simulink model "controller_dev_sg_HIL_noTP"  (R2018b)
settings: configuration reference "Physics" (kept outside this file)
model workspace (MAT data in the model file):
  m = 1000
values from neighbouring files (symbols this model uses):
  bool_activate_Vehicles : value not decoded    [controller_dev_sg.sldd]
  ModObj_ObjList_SendPort = 11004.0    [UDPPortConfig.sldd]
  ModSens_GpsSenDat_SendPort = 3002.0    [UDPPortConfig.sldd]
  sensors_freq_camera = 37.0    [controller_dev_sg.sldd]
  sensors_freq_gps = 20.0    [controller_dev_sg.sldd]
  sensors_freq_imu = 100.0    [controller_dev_sg.sldd]
  sensors_freq_lidar = 12.0    [controller_dev_sg.sldd]
  sensors_freq_radar = 20.0    [controller_dev_sg.sldd]
undefined symbols (not defined in the file or in its folder): activate_VariableFriction, C, tpa_map_Reference, tSPhysics, x0_vehiclepos_start_veh1, x0_vehiclepos_start_veh10, x0_vehiclepos_start_veh2, x0_vehiclepos_start_veh3, x0_vehiclepos_start_veh4, x0_vehiclepos_start_veh5, x0_vehiclepos_start_veh6, x0_vehiclepos_start_veh7, x0_vehiclepos_start_veh8, x0_vehiclepos_start_veh9
libraries: xpcutilitieslib x273, xpcrtudplib x215, aerolibconvert2 x48, simulink x30, etargetslib x26, speedgoatlib_IO612 x7, canmsglib x6, slrtlib x4
(part 13 of 16)

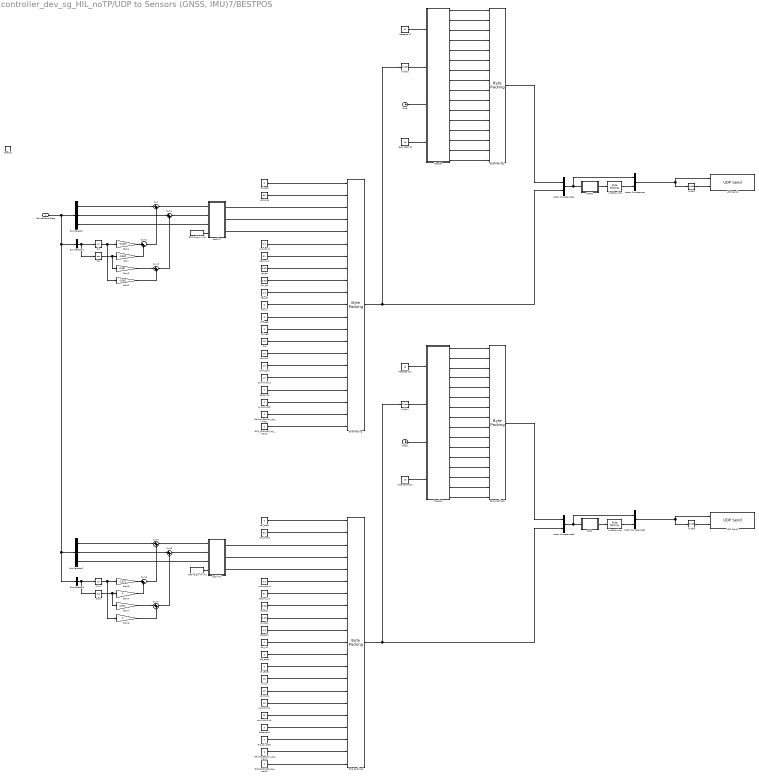
== system controller_dev_sg_HIL_noTP/UDP to Sensors (GNSS, IMU)7/BESTPOS ==
  VehicleSensorData : Inport
  Enable : EnablePort
  Bus Selector : BusSelector  OutputSignals=x_Loc1_m,y_Loc1_m,z_Loc1_m
  Bus Selector1 : BusSelector  OutputSignals=psi_YawAngleLoc1_rad
  Bus Selector2 : BusSelector  OutputSignals=x_Loc1_m,y_Loc1_m,z_Loc1_m
  Bus Selector3 : BusSelector  OutputSignals=psi_YawAngleLoc1_rad
  Byte Packing{,1..3} (4 alike) : xpcutilitieslib/Byte Packing 
  CRC1 : MATLAB Function  TreatAsAtomicUnit=on
  CRC32 : MATLAB Function  TreatAsAtomicUnit=on
  Clock : Clock
  Clock1 : Clock
  Cos : Trigonometry  Operator=cos
  Cos1 : Trigonometry  Operator=cos
  GPS Origin in llh : Constant  Value=[39.809786; -86.235148; 0.0]  OutDataTypeStr=double
  GPS Origin in llh1 : Constant  Value=[39.809786; -86.235148; 0.0]  OutDataTypeStr=double
  GPS_GLONASS_sig_mask1 : Constant  Value=0  OutDataTypeStr=uint8
  GPS_GLONASS_sig_mask2 : Constant  Value=0  OutDataTypeStr=uint8
  Gain : Gain  Gain=-0.502
  Gain1 : Gain  Gain=-0.457
  Gain2 : Gain  Gain=-0.502
  Gain3 : Gain  Gain=0.457
  Gain4 : Gain  Gain=0
  Gain5 : Gain  Gain=-1.571
  Gain6 : Gain  Gain=0
  Gain7 : Gain  Gain=1.571
  Galileo_BeiDou_sig_mask : Constant  Value=6  OutDataTypeStr=uint8
  Galileo_BeiDou_sig_mask1 : Constant  Value=6  OutDataTypeStr=uint8
  Header : MATLAB Function  TreatAsAtomicUnit=on
  Header1 : MATLAB Function  TreatAsAtomicUnit=on
  Message ID : Constant  Value=42  OutDataTypeStr=uint16
  Message ID1 : Constant  Value=42  OutDataTypeStr=uint16
  Reserved : Constant  Value=0  OutDataTypeStr=uint8
  Reserved1 : Constant  Value=0  OutDataTypeStr=uint8
  SVs : Constant  Value=19  OutDataTypeStr=uint8
  SVs1 : Constant  Value=19  OutDataTypeStr=uint8
  Sin : Trigonometry
  Sin1 : Trigonometry
  Sum{,1..7} (8 alike) : Sum  Inputs=|++
  UDP Send1 : xpcrtudplib/UDP Send  ipAddressVal=10.0.0.20  localPort=40681  toAddress=10.0.0.18  toPort=ModSens_GpsSenDat_SendPort  sampleTime=-1
      settings: SourceProductName=Simulink Real-Time  SourceProductBaseCode=XP
  UDP Send2 : xpcrtudplib/UDP Send  ipAddressVal=10.0.0.20  localPort=40781  toAddress=10.0.0.18  toPort=ModSens_GpsSenDat_SendPort + 1  sampleTime=-1
      settings: SourceProductName=Simulink Real-Time  SourceProductBaseCode=XP
  Vector Concatenate{,1..3} (4 alike) : Concatenate
  Width{1..4} (4 alike) : Width
  datum_id : Constant  Value=61  OutDataTypeStr=uint32
  datum_id1 : Constant  Value=61  OutDataTypeStr=uint32
  diff_age : Constant  Value=0  OutDataTypeStr=single
  diff_age1 : Constant  Value=0  OutDataTypeStr=single
  ext_sol_stat : Constant  Value=0  OutDataTypeStr=uint8
  ext_sol_stat1 : Constant  Value=0  OutDataTypeStr=uint8
  hgt_std : Constant  Value=1.0  OutDataTypeStr=single
  hgt_std1 : Constant  Value=1.0  OutDataTypeStr=single
  lat_std : Constant  Value=0.05  OutDataTypeStr=single
  lat_std1 : Constant  Value=0.05  OutDataTypeStr=single
  leap seconds : Constant  Value=19  OutDataTypeStr=single
  leap seconds1 : Constant  Value=19  OutDataTypeStr=single
  lon_std : Constant  Value=0.05  OutDataTypeStr=single
  lon_std1 : Constant  Value=0.05  OutDataTypeStr=single
  pos_type : Constant  Value=50  OutDataTypeStr=uint32
  pos_type1 : Constant  Value=50  OutDataTypeStr=uint32
  sol_age : Constant  Value=0  OutDataTypeStr=single
  sol_age1 : Constant  Value=0  OutDataTypeStr=single
  sol_stat : Constant  Value=0  OutDataTypeStr=uint32
  sol_stat1 : Constant  Value=0  OutDataTypeStr=uint32
  solnL1SVs : Constant  Value=19  OutDataTypeStr=uint8
  solnL1SVs1 : Constant  Value=19  OutDataTypeStr=uint8
  solnMultiSVs : Constant  Value=19  OutDataTypeStr=uint8
  solnMultiSVs1 : Constant  Value=19  OutDataTypeStr=uint8
  solnSVs : Constant  Value=19  OutDataTypeStr=uint8
  solnSVs1 : Constant  Value=19  OutDataTypeStr=uint8
  stn_id : Constant  Value=0  OutDataTypeStr=uint32
  stn_id1 : Constant  Value=0  OutDataTypeStr=uint32
  tcs2llhT : MATLAB Function  TreatAsAtomicUnit=on
  tcs2llhT1 : MATLAB Function  TreatAsAtomicUnit=on
  uint32touint1 : xpcutilitieslib/Byte Packing   MaskPackedDataType=uint8  MaskUnpackedDataTypes={'uint32'}  MaskAlignment=1
  uint32touint8 : xpcutilitieslib/Byte Packing   MaskPackedDataType=uint8  MaskUnpackedDataTypes={'uint32'}  MaskAlignment=1
  undulation : Constant  Value=0.0  OutDataTypeStr=single
  undulation1 : Constant  Value=0.0  OutDataTypeStr=single
  wires:
  CRC32/1(crc) -> uint32touint8/1
  uint32touint8/1 -> Vector Concatenate/2
  sol_stat/1 -> Byte Packing/1
  pos_type/1 -> Byte Packing/2
  undulation/1 -> Byte Packing/6
  datum_id/1 -> Byte Packing/7
  lat_std/1 -> Byte Packing/8
  lon_std/1 -> Byte Packing/9
  hgt_std/1 -> Byte Packing/10
  stn_id/1 -> Byte Packing/11
  diff_age/1 -> Byte Packing/12
  sol_age/1 -> Byte Packing/13
  SVs/1 -> Byte Packing/14
  solnSVs/1 -> Byte Packing/15
  solnL1SVs/1 -> Byte Packing/16
  solnMultiSVs/1 -> Byte Packing/17
  Reserved/1 -> Byte Packing/18
  ext_sol_stat/1 -> Byte Packing/19
  Galileo_BeiDou_sig_mask/1 -> Byte Packing/20
  GPS_GLONASS_sig_mask1/1 -> Byte Packing/21
  Header/1(first) -> Byte Packing1/1
  Header/2(second) -> Byte Packing1/2
  Header/3(third) -> Byte Packing1/3
  Header/4(hlength) -> Byte Packing1/4
  Header/5(id) -> Byte Packing1/5
  Header/6(type) -> Byte Packing1/6
  Header/7(port) -> Byte Packing1/7
  Header/8(mlength) -> Byte Packing1/8
  Header/9(seq) -> Byte Packing1/9
  Header/10(idletime) -> Byte Packing1/10
  Header/11(timestatus) -> Byte Packing1/11
  Header/12(week) -> Byte Packing1/12
  Header/13(ms) -> Byte Packing1/13
  Header/14(recstatus) -> Byte Packing1/14
  Header/15(reserved) -> Byte Packing1/15
  Header/16(version) -> Byte Packing1/16
  Message ID/1 -> Header/1("id ")
  Width2/1 -> Header/2(length)
  leap seconds/1 -> Header/4(leapseconds)
  Clock/1 -> Header/3(time)
  Vector Concatenate1/1 -> Vector Concatenate/1, CRC32/1(data)
  Byte Packing1/1 -> Vector Concatenate1/1
  Byte Packing/1 -> Width2/1, Vector Concatenate1/2
  Bus Selector/3 -> tcs2llhT/3(z)  "<z_Loc1_m>"
  tcs2llhT/1(lat) -> Byte Packing/3
  tcs2llhT/2(lon) -> Byte Packing/4
  tcs2llhT/3(hgt) -> Byte Packing/5
  GPS Origin in llh/1 -> tcs2llhT/4(origin)
  Width1/1 -> UDP Send1/2
  Vector Concatenate/1 -> UDP Send1/1, Width1/1
  Bus Selector/1 -> Sum/1  "<x_Loc1_m>"
  Bus Selector/2 -> Sum1/1  "<y_Loc1_m>"
  Sum1/1 -> tcs2llhT/2(y)
  Sum/1 -> tcs2llhT/1(x)
  Bus Selector1/1 -> Cos/1, Sin/1  "<psi_YawAngleLoc1_rad>"
  Cos/1 -> Gain3/1, Gain/1
  Sin/1 -> Gain2/1, Gain1/1
  Gain1/1 -> Sum2/1
  Gain/1 -> Sum2/2
  Sum2/1 -> Sum/2
  Gain2/1 -> Sum3/2
  Gain3/1 -> Sum3/1
  Sum3/1 -> Sum1/2
  Sum7/1 -> Sum5/2
  Gain4/1 -> Sum6/2
  Gain5/1 -> Sum6/1
  Sum6/1 -> Sum4/2
  Sin1/1 -> Gain6/1, Gain5/1
  Cos1/1 -> Gain7/1, Gain4/1
  Bus Selector3/1 -> Cos1/1, Sin1/1  "<psi_YawAngleLoc1_rad>"
  Header1/1(first) -> Byte Packing3/1
  lon_std1/1 -> Byte Packing2/9
  Header1/10(idletime) -> Byte Packing3/10
  tcs2llhT1/2(lon) -> Byte Packing2/4
  Header1/8(mlength) -> Byte Packing3/8
  tcs2llhT1/3(hgt) -> Byte Packing2/5
  tcs2llhT1/1(lat) -> Byte Packing2/3
  Header1/5(id) -> Byte Packing3/5
  undulation1/1 -> Byte Packing2/6
  Header1/9(seq) -> Byte Packing3/9
  Width4/1 -> Header1/2(length)
  Byte Packing2/1 -> Width4/1, Vector Concatenate3/2
  GPS Origin in llh1/1 -> tcs2llhT1/4(origin)
  Header1/2(second) -> Byte Packing3/2
  Header1/4(hlength) -> Byte Packing3/4
  Header1/3(third) -> Byte Packing3/3
  Header1/16(version) -> Byte Packing3/16
  Header1/6(type) -> Byte Packing3/6
  SVs1/1 -> Byte Packing2/14
  datum_id1/1 -> Byte Packing2/7
  Vector Concatenate3/1 -> Vector Concatenate2/1, CRC1/1(data)
  Clock1/1 -> Header1/3(time)
  Header1/11(timestatus) -> Byte Packing3/11
  leap seconds1/1 -> Header1/4(leapseconds)
  Header1/7(port) -> Byte Packing3/7
  stn_id1/1 -> Byte Packing2/11
  VehicleSensorData/1 -> Bus Selector3/1, Bus Selector2/1, Bus Selector1/1, Bus Selector/1
  lat_std1/1 -> Byte Packing2/8
  solnMultiSVs1/1 -> Byte Packing2/17
  pos_type1/1 -> Byte Packing2/2
  Vector Concatenate2/1 -> UDP Send2/1, Width3/1
  solnL1SVs1/1 -> Byte Packing2/16
  Bus Selector2/3 -> tcs2llhT1/3(z)  "<z_Loc1_m>"
  solnSVs1/1 -> Byte Packing2/15
  Message ID1/1 -> Header1/1("id ")
  Header1/15(reserved) -> Byte Packing3/15
  sol_age1/1 -> Byte Packing2/13
  Header1/12(week) -> Byte Packing3/12
  uint32touint1/1 -> Vector Concatenate2/2
  CRC1/1(crc) -> uint32touint1/1
  GPS_GLONASS_sig_mask2/1 -> Byte Packing2/21
  Byte Packing3/1 -> Vector Concatenate3/1
  Reserved1/1 -> Byte Packing2/18
  Sum5/1 -> tcs2llhT1/2(y)
  Header1/14(recstatus) -> Byte Packing3/14
  diff_age1/1 -> Byte Packing2/12
  sol_stat1/1 -> Byte Packing2/1
  Header1/13(ms) -> Byte Packing3/13
  Galileo_BeiDou_sig_mask1/1 -> Byte Packing2/20
  Bus Selector2/2 -> Sum5/1  "<y_Loc1_m>"
  Gain7/1 -> Sum7/1
  Sum4/1 -> tcs2llhT1/1(x)
  Bus Selector2/1 -> Sum4/1  "<x_Loc1_m>"
  Gain6/1 -> Sum7/2
  ext_sol_stat1/1 -> Byte Packing2/19
  hgt_std1/1 -> Byte Packing2/10
  Width3/1 -> UDP Send2/2

== system controller_dev_sg_HIL_noTP/UDP to Sensors (GNSS, IMU)7/BESTUTM ==
  VehicleSensorData : Inport
  Enable : EnablePort
  Bus Selector : BusSelector  OutputSignals=x_Loc1_m,y_Loc1_m,z_Loc1_m
  Byte Packing : xpcutilitieslib/Byte Packing   MaskPackedDataType=uint8  MaskUnpackedDataTypes={'uint32', 'uint32', 'uint32', 'uint32', 'double', 'double', 'double', 'single', 'uint32', 'single', 'single', 'single', 'uint32', 'single', 'single', 'uint8', 'uint8', 'uint8', 'uint8', 'uint8', 'uint8', 'uint8', 'uint8'}  MaskAlignment=1
  Byte Packing1 : xpcutilitieslib/Byte Packing   MaskPackedDataType=uint8  MaskUnpackedDataTypes={'uint8', 'uint8', 'uint8', 'uint8', 'uint16', 'uint8', 'uint8', 'uint16', 'uint16', 'uint8', 'uint8', 'uint16', 'uint32', 'uint32', 'uint16', 'uint16'}  MaskAlignment=1
  CRC32 : MATLAB Function  TreatAsAtomicUnit=on
  Clock : Clock
  Data Type Conversion : DataTypeConversion  OutDataTypeStr=uint32
  Data Type Conversion1 : DataTypeConversion  OutDataTypeStr=uint32
  GPS Origin in llh : Constant  Value=[39.809786; -86.235148; 0.0]  OutDataTypeStr=double
  GPS_GLONASS_sig_mask1 : Constant  Value=0  OutDataTypeStr=uint8
  Galileo_BeiDou_sig_mask : Constant  Value=6  OutDataTypeStr=uint8
  Header : MATLAB Function  TreatAsAtomicUnit=on
  MATLAB Function : MATLAB Function  TreatAsAtomicUnit=on
  Message ID : Constant  Value=726  OutDataTypeStr=uint16
  Reserved : Constant  Value=0  OutDataTypeStr=uint8
  SVs : Constant  Value=19  OutDataTypeStr=uint8
  UDP Send1 : xpcrtudplib/UDP Send  ipAddressVal=10.0.0.20  localPort=40785  toAddress=10.0.0.18  toPort=ModSens_GpsSenDat_SendPort + 1  sampleTime=-1
      settings: SourceProductName=Simulink Real-Time  SourceProductBaseCode=XP
  UDP Send5 : xpcrtudplib/UDP Send  ipAddressVal=10.0.0.20  localPort=40685  toAddress=10.0.0.18  toPort=ModSens_GpsSenDat_SendPort  sampleTime=-1
      settings: SourceProductName=Simulink Real-Time  SourceProductBaseCode=XP
  Vector Concatenate : Concatenate
  Vector Concatenate1 : Concatenate
  Width2 : Width
  Width5 : Width
  datum id : Constant  Value=61  OutDataTypeStr=uint32
  diff_age : Constant  Value=0  OutDataTypeStr=single
  e std : Constant  Value=0  OutDataTypeStr=single
  ext sol stat : Constant  Value=0  OutDataTypeStr=uint8
  ggL1 : Constant  Value=19  OutDataTypeStr=uint8
  hgt std : Constant  Value=0  OutDataTypeStr=single
  leap seconds : Constant  Value=19  OutDataTypeStr=single
  n std : Constant  Value=0  OutDataTypeStr=single
  pos_type : Constant  Value=16  OutDataTypeStr=uint32
  sol_age : Constant  Value=0  OutDataTypeStr=single
  sol_stat : Constant  Value=0  OutDataTypeStr=uint32
  solnMultiSV : Constant  Value=19  OutDataTypeStr=uint8
  solnSVs : Constant  Value=19  OutDataTypeStr=uint8
  stn id : Constant  Value=0  OutDataTypeStr=uint32
  tcs2llhT : MATLAB Function  TreatAsAtomicUnit=on
  uint32touint8 : xpcutilitieslib/Byte Packing   MaskPackedDataType=uint8  MaskUnpackedDataTypes={'uint32'}  MaskAlignment=1
  undulation : Constant  Value=0.0  OutDataTypeStr=single
  wires:
  VehicleSensorData/1 -> Bus Selector/1
  CRC32/1(crc) -> uint32touint8/1
  uint32touint8/1 -> Vector Concatenate/2
  Message ID/1 -> Header/1("id ")
  Header/7(port) -> Byte Packing1/7
  Byte Packing1/1 -> Vector Concatenate1/1
  Header/9(seq) -> Byte Packing1/9
  Width2/1 -> Header/2(length)
  Header/12(week) -> Byte Packing1/12
  Header/1(first) -> Byte Packing1/1
  leap seconds/1 -> Header/4(leapseconds)
  Header/4(hlength) -> Byte Packing1/4
  Header/8(mlength) -> Byte Packing1/8
  Header/10(idletime) -> Byte Packing1/10
  Header/2(second) -> Byte Packing1/2
  Header/15(reserved) -> Byte Packing1/15
  Clock/1 -> Header/3(time)
  Header/14(recstatus) -> Byte Packing1/14
  Header/6(type) -> Byte Packing1/6
  Header/5(id) -> Byte Packing1/5
  Header/3(third) -> Byte Packing1/3
  Header/16(version) -> Byte Packing1/16
  Header/13(ms) -> Byte Packing1/13
  Header/11(timestatus) -> Byte Packing1/11
  sol_stat/1 -> Byte Packing/1
  pos_type/1 -> Byte Packing/2
  undulation/1 -> Byte Packing/8
  datum id/1 -> Byte Packing/9
  n std/1 -> Byte Packing/10
  e std/1 -> Byte Packing/11
  hgt std/1 -> Byte Packing/12
  stn id/1 -> Byte Packing/13
  diff_age/1 -> Byte Packing/14
  sol_age/1 -> Byte Packing/15
  SVs/1 -> Byte Packing/16
  solnSVs/1 -> Byte Packing/17
  ggL1/1 -> Byte Packing/18
  solnMultiSV/1 -> Byte Packing/19
  Reserved/1 -> Byte Packing/20
  ext sol stat/1 -> Byte Packing/21
  Galileo_BeiDou_sig_mask/1 -> Byte Packing/22
  GPS_GLONASS_sig_mask1/1 -> Byte Packing/23
  Vector Concatenate1/1 -> Vector Concatenate/1, CRC32/1(data)
  Byte Packing/1 -> Width2/1, Vector Concatenate1/2
  GPS Origin in llh/1 -> tcs2llhT/4(origin)
  tcs2llhT/3(hgt) -> Byte Packing/7
  Bus Selector/2 -> tcs2llhT/2(y)  "<y_Loc1_m>"
  Bus Selector/1 -> tcs2llhT/1(x)  "<x_Loc1_m>"
  Bus Selector/3 -> tcs2llhT/3(z)  "<z_Loc1_m>"
  tcs2llhT/1(lat) -> MATLAB Function/1(Lat)
  tcs2llhT/2(lon) -> MATLAB Function/2(Lon)
  MATLAB Function/1(zone_nbr) -> Data Type Conversion/1
  Data Type Conversion/1 -> Byte Packing/3
  MATLAB Function/2(zone_ltr) -> Data Type Conversion1/1
  Data Type Conversion1/1 -> Byte Packing/4
  MATLAB Function/3(northing) -> Byte Packing/5
  MATLAB Function/4(easting) -> Byte Packing/6
  Vector Concatenate/1 -> UDP Send1/1, UDP Send5/1, Width5/1
  Width5/1 -> UDP Send1/2, UDP Send5/2

== system controller_dev_sg_HIL_noTP/UDP to Sensors (GNSS, IMU)7/BESTVAL ==
  VehicleSensorData : Inport
  SimRealState : Inport  Port=2
  Enable : EnablePort
  Angle Conversion2 : aerolibconvert2/Angle Conversion  IU=rad  OU=deg
  Bus Selector : BusSelector  OutputSignals=vx_CoGVel1_mps,vy_CoGVel1_mps,x_Loc1_m,y_Loc1_m,z_Loc1_m
  Bus Selector1 : BusSelector  OutputSignals=psi_rad
  Byte Packing : xpcutilitieslib/Byte Packing   MaskPackedDataType=uint8  MaskUnpackedDataTypes={'uint32', 'uint32', 'single', 'single', 'double', 'double', 'double', 'single'}  MaskAlignment=1
  Byte Packing1 : xpcutilitieslib/Byte Packing   MaskPackedDataType=uint8  MaskUnpackedDataTypes={'uint8', 'uint8', 'uint8', 'uint8', 'uint16', 'uint8', 'uint8', 'uint16', 'uint16', 'uint8', 'uint8', 'uint16', 'uint32', 'uint32', 'uint16', 'uint16'}  MaskAlignment=1
  CRC32 : MATLAB Function  TreatAsAtomicUnit=on
  Clock : Clock
  GPS Origin in llh : Constant  Value=[39.809786; -86.235148; 0.0]  OutDataTypeStr=double
  Gain : Gain  Gain=-1
  Header : MATLAB Function  TreatAsAtomicUnit=on
  Message ID : Constant  Value=99  OutDataTypeStr=uint16
  Plus : Sum  AccumDataTypeStr=double
  Reserved : Constant  Value=0  OutDataTypeStr=single
  UDP Send1 : xpcrtudplib/UDP Send  ipAddressVal=10.0.0.20  localPort=40782  toAddress=10.0.0.18  toPort=ModSens_GpsSenDat_SendPort + 1  sampleTime=-1
      settings: SourceProductName=Simulink Real-Time  SourceProductBaseCode=XP
  UDP Send2 : xpcrtudplib/UDP Send  ipAddressVal=10.0.0.20  localPort=40682  toAddress=10.0.0.18  toPort=ModSens_GpsSenDat_SendPort  sampleTime=-1
      settings: SourceProductName=Simulink Real-Time  SourceProductBaseCode=XP
  Vector Concatenate : Concatenate
  Vector Concatenate1 : Concatenate
  Vector Concatenate2 : Concatenate
  Width1 : Width
  Width2 : Width
  age : Constant  Value=4  OutDataTypeStr=single
  grid conv angle : MATLAB Function  TreatAsAtomicUnit=on
  latency : Constant  Value=0.25  OutDataTypeStr=single
  leap seconds : Constant  Value=19  OutDataTypeStr=single
  norm : MATLAB Function  TreatAsAtomicUnit=on
  normalizeAngle360 : MATLAB Function  TreatAsAtomicUnit=on
  sol_stat : Constant  Value=0  OutDataTypeStr=uint32
  tcs2llhT : MATLAB Function  TreatAsAtomicUnit=on
  uint32touint8 : xpcutilitieslib/Byte Packing   MaskPackedDataType=uint8  MaskUnpackedDataTypes={'uint32'}  MaskAlignment=1
  vel_type : Constant  Value=17  OutDataTypeStr=uint32
  vert_spd : Constant  Value=0.0  OutDataTypeStr=double
  wires:
  VehicleSensorData/1 -> Bus Selector/1
  CRC32/1(crc) -> uint32touint8/1
  uint32touint8/1 -> Vector Concatenate/2
  Header/14(recstatus) -> Byte Packing1/14
  Header/15(reserved) -> Byte Packing1/15
  Header/16(version) -> Byte Packing1/16
  Header/13(ms) -> Byte Packing1/13
  Header/10(idletime) -> Byte Packing1/10
  Header/11(timestatus) -> Byte Packing1/11
  Clock/1 -> Header/3(time)
  Header/7(port) -> Byte Packing1/7
  Header/6(type) -> Byte Packing1/6
  Header/8(mlength) -> Byte Packing1/8
  Header/5(id) -> Byte Packing1/5
  Header/3(third) -> Byte Packing1/3
  Header/4(hlength) -> Byte Packing1/4
  Header/1(first) -> Byte Packing1/1
  leap seconds/1 -> Header/4(leapseconds)
  Message ID/1 -> Header/1("id ")
  Width2/1 -> Header/2(length)
  Header/2(second) -> Byte Packing1/2
  Header/12(week) -> Byte Packing1/12
  Byte Packing1/1 -> Vector Concatenate1/1
  Header/9(seq) -> Byte Packing1/9
  sol_stat/1 -> Byte Packing/1
  vel_type/1 -> Byte Packing/2
  latency/1 -> Byte Packing/3
  age/1 -> Byte Packing/4
  vert_spd/1 -> Byte Packing/7
  Reserved/1 -> Byte Packing/8
  Vector Concatenate1/1 -> Vector Concatenate/1, CRC32/1(data)
  Byte Packing/1 -> Width2/1, Vector Concatenate1/2
  Bus Selector/2 -> Vector Concatenate2/2  "<vy_CoGVel1_mps>"
  Bus Selector/1 -> Vector Concatenate2/1  "<vx_CoGVel1_mps>"
  Vector Concatenate2/1 -> norm/1(u)
  GPS Origin in llh/1 -> tcs2llhT/4(origin)
  Bus Selector/5 -> tcs2llhT/3(z)  "<z_Loc1_m>"
  Bus Selector/4 -> tcs2llhT/2(y)  "<y_Loc1_m>"
  Bus Selector/3 -> tcs2llhT/1(x)  "<x_Loc1_m>"
  tcs2llhT/1(lat) -> grid conv angle/1(lat)
  tcs2llhT/2(lon) -> grid conv angle/2(lon)
  norm/1(y) -> Byte Packing/5
  SimRealState/1 -> Bus Selector1/1
  Angle Conversion2/1 -> Gain/1
  Bus Selector1/1 -> Angle Conversion2/1  "<psi_rad>"
  Plus/1 -> normalizeAngle360/1(u)
  grid conv angle/1(gamma) -> Plus/1
  normalizeAngle360/1(y) -> Byte Packing/6
  Gain/1 -> Plus/2
  Vector Concatenate/1 -> Width1/1, UDP Send1/1, UDP Send2/1
  Width1/1 -> UDP Send1/2, UDP Send2/2

== system controller_dev_sg_HIL_noTP/UDP to Sensors (GNSS, IMU)7/CORRIMUDATA ==
  VehicleSensorData : Inport
  Enable : EnablePort
  Bus Selector : BusSelector  OutputSignals=dTheta_PitchRateIMU1_radps,dPhi_RollRateIMU1_radps,dPsi_YawRateIMU1_radps,ay_CoGIMU1_mps2,ax_CoGIMU1_mps2,az_CoGIMU1_mps2
  Byte Packing : xpcutilitieslib/Byte Packing   MaskPackedDataType=uint8  MaskUnpackedDataTypes={'uint32', 'double', 'double', 'double', 'double', 'double', 'double', 'double'}  MaskAlignment=1
  Byte Packing1 : xpcutilitieslib/Byte Packing   MaskPackedDataType=uint8  MaskUnpackedDataTypes={'uint8', 'uint8', 'uint8', 'uint8', 'uint16', 'uint8', 'uint8', 'uint16', 'uint16', 'uint8', 'uint8', 'uint16', 'uint32', 'uint32', 'uint16', 'uint16'}  MaskAlignment=1
  CRC32 : MATLAB Function  TreatAsAtomicUnit=on
  Clock : Clock
  Clock1 : Clock
  GNSS Week : Constant  Value=1900  OutDataTypeStr=uint32
  Header : MATLAB Function  TreatAsAtomicUnit=on
  Message ID : Constant  Value=812  OutDataTypeStr=uint16
  UDP Send1 : xpcrtudplib/UDP Send  ipAddressVal=10.0.0.20  localPort=40783  toAddress=10.0.0.18  toPort=ModSens_GpsSenDat_SendPort + 1  sampleTime=-1
      settings: SourceProductName=Simulink Real-Time  SourceProductBaseCode=XP
  UDP Send3 : xpcrtudplib/UDP Send  ipAddressVal=10.0.0.20  localPort=40683  toAddress=10.0.0.18  toPort=ModSens_GpsSenDat_SendPort  sampleTime=-1
      settings: SourceProductName=Simulink Real-Time  SourceProductBaseCode=XP
  Vector Concatenate : Concatenate
  Vector Concatenate1 : Concatenate
  Width2 : Width
  Width3 : Width
  leap seconds : Constant  Value=19  OutDataTypeStr=single
  uint32touint8 : xpcutilitieslib/Byte Packing   MaskPackedDataType=uint8  MaskUnpackedDataTypes={'uint32'}  MaskAlignment=1
  wires:
  VehicleSensorData/1 -> Bus Selector/1
  CRC32/1(crc) -> uint32touint8/1
  uint32touint8/1 -> Vector Concatenate/2
  Message ID/1 -> Header/1("id ")
  Header/9(seq) -> Byte Packing1/9
  Byte Packing1/1 -> Vector Concatenate1/1
  Header/12(week) -> Byte Packing1/12
  Width2/1 -> Header/2(length)
  leap seconds/1 -> Header/4(leapseconds)
  Header/2(second) -> Byte Packing1/2
  Header/6(type) -> Byte Packing1/6
  Header/4(hlength) -> Byte Packing1/4
  Header/8(mlength) -> Byte Packing1/8
  Header/5(id) -> Byte Packing1/5
  Header/1(first) -> Byte Packing1/1
  Header/3(third) -> Byte Packing1/3
  Header/16(version) -> Byte Packing1/16
  Header/11(timestatus) -> Byte Packing1/11
  Header/13(ms) -> Byte Packing1/13
  Header/10(idletime) -> Byte Packing1/10
  Header/15(reserved) -> Byte Packing1/15
  Header/14(recstatus) -> Byte Packing1/14
  Header/7(port) -> Byte Packing1/7
  Clock/1 -> Header/3(time)
  GNSS Week/1 -> Byte Packing/1
  Clock1/1 -> Byte Packing/2
  Vector Concatenate1/1 -> Vector Concatenate/1, CRC32/1(data)
  Byte Packing/1 -> Vector Concatenate1/2, Width2/1
  Bus Selector/1 -> Byte Packing/3  "<dTheta_PitchRateIMU1_radps>"
  Bus Selector/2 -> Byte Packing/4  "<dPhi_RollRateIMU1_radps>"
  Bus Selector/3 -> Byte Packing/5  "<dPsi_YawRateIMU1_radps>"
  Bus Selector/6 -> Byte Packing/8  "<az_CoGIMU1_mps2>"
  Bus Selector/4 -> Byte Packing/6  "<ay_CoGIMU1_mps2>"
  Bus Selector/5 -> Byte Packing/7  "<ax_CoGIMU1_mps2>"
  Width3/1 -> UDP Send1/2, UDP Send3/2
  Vector Concatenate/1 -> UDP Send1/1, UDP Send3/1, Width3/1

== system controller_dev_sg_HIL_noTP/UDP to Sensors (GNSS, IMU)7/DUALANTENNAHEADING ==
  VehicleSensorData : Inport
  SimRealState : Inport  Port=2
  Enable : EnablePort
  Angle Conversion{1..4} (4 alike) : aerolibconvert2/Angle Conversion  IU=rad  OU=deg
  Bus Selector : BusSelector  OutputSignals=x_Loc1_m,y_Loc1_m,z_Loc1_m,theta_PitchAngleLoc1_rad
  Bus Selector1 : BusSelector  OutputSignals=psi_rad
  Bus Selector2 : BusSelector  OutputSignals=x_Loc1_m,y_Loc1_m,z_Loc1_m,theta_PitchAngleLoc1_rad
  Bus Selector3 : BusSelector  OutputSignals=psi_rad
  Byte Packing{,1..3} (4 alike) : xpcutilitieslib/Byte Packing 
  CRC1 : MATLAB Function  TreatAsAtomicUnit=on
  CRC32 : MATLAB Function  TreatAsAtomicUnit=on
  Clock : Clock
  Clock1 : Clock
  Constant : Constant  Value=90  OutDataTypeStr=double
  Constant1 : Constant  Value=180  OutDataTypeStr=double
  Data Type Conversion{1..3,7} (4 alike) : DataTypeConversion  OutDataTypeStr=single
  GPS Origin in llh : Constant  Value=[39.809786; -86.235148; 0.0]  OutDataTypeStr=double
  GPS Origin in llh1 : Constant  Value=[39.809786; -86.235148; 0.0]  OutDataTypeStr=double
  GPS_GLONASS_sig_mask1 : Constant  Value=0  OutDataTypeStr=uint8
  GPS_GLONASS_sig_mask2 : Constant  Value=0  OutDataTypeStr=uint8
  Gain : Gain  Gain=-1
  Gain1 : Gain  Gain=-1
  Galileo_BeiDou_sig_mask : Constant  Value=6  OutDataTypeStr=uint8
  Galileo_BeiDou_sig_mask1 : Constant  Value=6  OutDataTypeStr=uint8
  Header : MATLAB Function  TreatAsAtomicUnit=on
  Header1 : MATLAB Function  TreatAsAtomicUnit=on
  Message ID : Constant  Value=2042  OutDataTypeStr=uint16
  Message ID1 : Constant  Value=2042  OutDataTypeStr=uint16
  Plus{,1..3} (4 alike) : Sum  AccumDataTypeStr=double
  Reserved : Constant  Value=0  OutDataTypeStr=single
  Reserved1 : Constant  Value=0  OutDataTypeStr=single
  SVs : Constant  Value=19  OutDataTypeStr=uint8
  SVs1 : Constant  Value=19  OutDataTypeStr=uint8
  UDP Send2 : xpcrtudplib/UDP Send  ipAddressVal=10.0.0.20  localPort=40788  toAddress=10.0.0.18  toPort=ModSens_GpsSenDat_SendPort + 1  sampleTime=-1
      settings: SourceProductName=Simulink Real-Time  SourceProductBaseCode=XP
  UDP Send3 : xpcrtudplib/UDP Send  ipAddressVal=10.0.0.20  localPort=40688  toAddress=10.0.0.18  toPort=ModSens_GpsSenDat_SendPort  sampleTime=-1
      settings: SourceProductName=Simulink Real-Time  SourceProductBaseCode=XP
  Vector Concatenate{,1..3} (4 alike) : Concatenate
  Width{1..4} (4 alike) : Width
  ext_sol_stat : Constant  Value=0  OutDataTypeStr=uint8
  ext_sol_stat1 : Constant  Value=0  OutDataTypeStr=uint8
  grid conv angle : MATLAB Function  TreatAsAtomicUnit=on
  grid conv angle1 : MATLAB Function  TreatAsAtomicUnit=on
  hdg std dev : Constant  Value=0  OutDataTypeStr=single
  hdg std dev1 : Constant  Value=0  OutDataTypeStr=single
  leap seconds : Constant  Value=19  OutDataTypeStr=single
  leap seconds1 : Constant  Value=19  OutDataTypeStr=single
  length : Constant  Value=-1  OutDataTypeStr=single
  length1 : Constant  Value=-1  OutDataTypeStr=single
  multi : Constant  Value=0  OutDataTypeStr=uint8
  multi1 : Constant  Value=0  OutDataTypeStr=uint8
  normalizeAngle1 : MATLAB Function  TreatAsAtomicUnit=on
  normalizeAngle360 : MATLAB Function  TreatAsAtomicUnit=on
  obs : Constant  Value=0  OutDataTypeStr=uint8
  obs1 : Constant  Value=0  OutDataTypeStr=uint8
  pos_type : Constant  Value=50  OutDataTypeStr=uint32
  pos_type1 : Constant  Value=50  OutDataTypeStr=uint32
  ptch std dev1 : Constant  Value=0  OutDataTypeStr=single
  ptch std dev2 : Constant  Value=0  OutDataTypeStr=single
  sol source : Constant  Value=0  OutDataTypeStr=uint8
  sol source1 : Constant  Value=0  OutDataTypeStr=uint8
  sol_stat : Constant  Value=0  OutDataTypeStr=uint32
  sol_stat1 : Constant  Value=0  OutDataTypeStr=uint32
  solnSVs : Constant  Value=19  OutDataTypeStr=uint8
  solnSVs1 : Constant  Value=19  OutDataTypeStr=uint8
  stn_id : Constant  Value=0  OutDataTypeStr=uint32
  stn_id1 : Constant  Value=0  OutDataTypeStr=uint32
  tcs2llhT : MATLAB Function  TreatAsAtomicUnit=on
  tcs2llhT1 : MATLAB Function  TreatAsAtomicUnit=on
  uint32touint1 : xpcutilitieslib/Byte Packing   MaskPackedDataType=uint8  MaskUnpackedDataTypes={'uint32'}  MaskAlignment=1
  uint32touint8 : xpcutilitieslib/Byte Packing   MaskPackedDataType=uint8  MaskUnpackedDataTypes={'uint32'}  MaskAlignment=1
  wires:
  CRC32/1(crc) -> uint32touint8/1
  uint32touint8/1 -> Vector Concatenate/2
  Vector Concatenate1/1 -> Vector Concatenate/1, CRC32/1(data)
  Width3/1 -> UDP Send3/2
  Vector Concatenate/1 -> UDP Send3/1, Width3/1
  Header/10(idletime) -> Byte Packing1/10
  Header/16(version) -> Byte Packing1/16
  Header/7(port) -> Byte Packing1/7
  Header/11(timestatus) -> Byte Packing1/11
  Header/8(mlength) -> Byte Packing1/8
  Header/12(week) -> Byte Packing1/12
  leap seconds/1 -> Header/4(leapseconds)
  Byte Packing1/1 -> Vector Concatenate1/1
  Header/6(type) -> Byte Packing1/6
  Header/9(seq) -> Byte Packing1/9
  Header/5(id) -> Byte Packing1/5
  Header/1(first) -> Byte Packing1/1
  Message ID/1 -> Header/1("id ")
  Width2/1 -> Header/2(length)
  Header/3(third) -> Byte Packing1/3
  Header/4(hlength) -> Byte Packing1/4
  Clock/1 -> Header/3(time)
  Header/2(second) -> Byte Packing1/2
  Header/15(reserved) -> Byte Packing1/15
  Byte Packing/1 -> Vector Concatenate1/2, Width2/1
  Header/14(recstatus) -> Byte Packing1/14
  Header/13(ms) -> Byte Packing1/13
  Bus Selector1/1 -> Angle Conversion2/1  "<psi_rad>"
  Angle Conversion2/1 -> Gain/1
  tcs2llhT/2(lon) -> grid conv angle/2(lon)
  tcs2llhT/1(lat) -> grid conv angle/1(lat)
  grid conv angle/1(gamma) -> Plus/1
  GPS Origin in llh/1 -> tcs2llhT/4(origin)
  sol_stat/1 -> Byte Packing/1
  pos_type/1 -> Byte Packing/2
  length/1 -> Byte Packing/3
  Gain/1 -> Plus/2
  Bus Selector/1 -> tcs2llhT/1(x)  "<x_Loc1_m>"
  Bus Selector/2 -> tcs2llhT/2(y)  "<y_Loc1_m>"
  Bus Selector/3 -> tcs2llhT/3(z)  "<z_Loc1_m>"
  normalizeAngle360/1(y) -> Data Type Conversion1/1
  Bus Selector/4 -> Angle Conversion1/1  "<theta_PitchAngleLoc1_rad>"
  Angle Conversion1/1 -> Data Type Conversion7/1
  Reserved/1 -> Byte Packing/6
  hdg std dev/1 -> Byte Packing/7
  ptch std dev1/1 -> Byte Packing/8
  stn_id/1 -> Byte Packing/9
  SVs/1 -> Byte Packing/10
  solnSVs/1 -> Byte Packing/11
  obs/1 -> Byte Packing/12
  multi/1 -> Byte Packing/13
  sol source/1 -> Byte Packing/14
  ext_sol_stat/1 -> Byte Packing/15
  Galileo_BeiDou_sig_mask/1 -> Byte Packing/16
  GPS_GLONASS_sig_mask1/1 -> Byte Packing/17
  Data Type Conversion7/1 -> Byte Packing/5
  Data Type Conversion1/1 -> Byte Packing/4
  Angle Conversion4/1 -> Gain1/1
  sol source1/1 -> Byte Packing2/14
  Header1/6(type) -> Byte Packing3/6
  CRC1/1(crc) -> uint32touint1/1
  Data Type Conversion2/1 -> Byte Packing2/4
  obs1/1 -> Byte Packing2/12
  Bus Selector2/2 -> tcs2llhT1/2(y)  "<y_Loc1_m>"
  Bus Selector2/4 -> Angle Conversion3/1  "<theta_PitchAngleLoc1_rad>"
  tcs2llhT1/1(lat) -> grid conv angle1/1(lat)
  Reserved1/1 -> Byte Packing2/6
  tcs2llhT1/2(lon) -> grid conv angle1/2(lon)
  Bus Selector3/1 -> Angle Conversion4/1  "<psi_rad>"
  SimRealState/1 -> Bus Selector3/1, Bus Selector1/1
  normalizeAngle1/1(y) -> Data Type Conversion2/1
  Header1/2(second) -> Byte Packing3/2
  stn_id1/1 -> Byte Packing2/9
  Header1/3(third) -> Byte Packing3/3
  VehicleSensorData/1 -> Bus Selector2/1, Bus Selector/1
  Bus Selector2/3 -> tcs2llhT1/3(z)  "<z_Loc1_m>"
  Byte Packing3/1 -> Vector Concatenate3/1
  SVs1/1 -> Byte Packing2/10
  Gain1/1 -> Plus1/2
  length1/1 -> Byte Packing2/3
  sol_stat1/1 -> Byte Packing2/1
  Bus Selector2/1 -> tcs2llhT1/1(x)  "<x_Loc1_m>"
  GPS Origin in llh1/1 -> tcs2llhT1/4(origin)
  solnSVs1/1 -> Byte Packing2/11
  GPS_GLONASS_sig_mask2/1 -> Byte Packing2/17
  Galileo_BeiDou_sig_mask1/1 -> Byte Packing2/16
  grid conv angle1/1(gamma) -> Plus1/1
  Header1/14(recstatus) -> Byte Packing3/14
  Byte Packing2/1 -> Vector Concatenate3/2, Width1/1
  ptch std dev2/1 -> Byte Packing2/8
  pos_type1/1 -> Byte Packing2/2
  Header1/13(ms) -> Byte Packing3/13
  multi1/1 -> Byte Packing2/13
  Header1/15(reserved) -> Byte Packing3/15
  Header1/16(version) -> Byte Packing3/16
  Header1/7(port) -> Byte Packing3/7
  Angle Conversion3/1 -> Data Type Conversion3/1
  Header1/8(mlength) -> Byte Packing3/8
  leap seconds1/1 -> Header1/4(leapseconds)
  Header1/4(hlength) -> Byte Packing3/4
  hdg std dev1/1 -> Byte Packing2/7
  Header1/1(first) -> Byte Packing3/1
  Header1/12(week) -> Byte Packing3/12
  Data Type Conversion3/1 -> Byte Packing2/5
  ext_sol_stat1/1 -> Byte Packing2/15
  Vector Concatenate3/1 -> Vector Concatenate2/1, CRC1/1(data)
  Header1/5(id) -> Byte Packing3/5
  Header1/9(seq) -> Byte Packing3/9
  Vector Concatenate2/1 -> UDP Send2/1, Width4/1
  Header1/10(idletime) -> Byte Packing3/10
  Clock1/1 -> Header1/3(time)
  Width1/1 -> Header1/2(length)
  Message ID1/1 -> Header1/1("id ")
  Width4/1 -> UDP Send2/2
  Header1/11(timestatus) -> Byte Packing3/11
  uint32touint1/1 -> Vector Concatenate2/2
  Plus2/1 -> normalizeAngle360/1(u)
  Plus/1 -> Plus2/2
  Constant/1 -> Plus2/1
  Constant1/1 -> Plus3/1
  Plus1/1 -> Plus3/2
  Plus3/1 -> normalizeAngle1/1(u)

== system controller_dev_sg_HIL_noTP/UDP to Sensors (GNSS, IMU)7/INSPVA ==
  VehicleSensorData : Inport
  SimRealState : Inport  Port=2
  Enable : EnablePort
  Angle Conversion2 : aerolibconvert2/Angle Conversion  IU=rad  OU=deg
  Bus Selector : BusSelector  OutputSignals=x_Loc1_m,y_Loc1_m,z_Loc1_m,vx_CoGVel1_mps,vy_CoGVel1_mps,dPhi_RollRateIMU1_radps,dTheta_PitchRateIMU1_radps
  Bus Selector1 : BusSelector  OutputSignals=psi_rad
  Byte Packing : xpcutilitieslib/Byte Packing   MaskPackedDataType=uint8  MaskUnpackedDataTypes={'uint32', 'double', 'double', 'double', 'double', 'double', 'double', 'double', 'double', 'double', 'double', 'uint32'}  MaskAlignment=1
  Byte Packing1 : xpcutilitieslib/Byte Packing   MaskPackedDataType=uint8  MaskUnpackedDataTypes={'uint8', 'uint8', 'uint8', 'uint8', 'uint16', 'uint8', 'uint8', 'uint16', 'uint16', 'uint8', 'uint8', 'uint16', 'uint32', 'uint32', 'uint16', 'uint16'}  MaskAlignment=1
  CRC32 : MATLAB Function  TreatAsAtomicUnit=on
  Clock : Clock
  Clock1 : Clock
  Constant : Constant  Value=3  OutDataTypeStr=uint32
  Constant1 : Constant  Value=0  OutDataTypeStr=double
  GNSS Week : Constant  Value=1900  OutDataTypeStr=uint32
  GPS Origin in llh : Constant  Value=[39.809786; -86.235148; 0.0]  OutDataTypeStr=double
  Gain : Gain  Gain=-1
  Header : MATLAB Function  TreatAsAtomicUnit=on
  Message ID : Constant  Value=507  OutDataTypeStr=uint16
  Plus : Sum  AccumDataTypeStr=double
  UDP Send1 : xpcrtudplib/UDP Send  ipAddressVal=10.0.0.20  localPort=40786  toAddress=10.0.0.18  toPort=ModSens_GpsSenDat_SendPort + 1  sampleTime=-1
      settings: SourceProductName=Simulink Real-Time  SourceProductBaseCode=XP
  UDP Send5 : xpcrtudplib/UDP Send  ipAddressVal=10.0.0.20  localPort=40686  toAddress=10.0.0.18  toPort=ModSens_GpsSenDat_SendPort  sampleTime=-1
      settings: SourceProductName=Simulink Real-Time  SourceProductBaseCode=XP
  Vector Concatenate : Concatenate
  Vector Concatenate1 : Concatenate
  Width2 : Width
  Width5 : Width
  grid conv angle : MATLAB Function  TreatAsAtomicUnit=on
  leap seconds : Constant  Value=19  OutDataTypeStr=single
  normalizeAngle360 : MATLAB Function  TreatAsAtomicUnit=on
  tcs2llhT : MATLAB Function  TreatAsAtomicUnit=on
  uint32touint8 : xpcutilitieslib/Byte Packing   MaskPackedDataType=uint8  MaskUnpackedDataTypes={'uint32'}  MaskAlignment=1
  wires:
  VehicleSensorData/1 -> Bus Selector/1
  CRC32/1(crc) -> uint32touint8/1
  uint32touint8/1 -> Vector Concatenate/2
  Message ID/1 -> Header/1("id ")
  Header/7(port) -> Byte Packing1/7
  Byte Packing1/1 -> Vector Concatenate1/1
  Header/9(seq) -> Byte Packing1/9
  Width2/1 -> Header/2(length)
  Header/12(week) -> Byte Packing1/12
  Header/1(first) -> Byte Packing1/1
  leap seconds/1 -> Header/4(leapseconds)
  Header/4(hlength) -> Byte Packing1/4
  Header/8(mlength) -> Byte Packing1/8
  Header/10(idletime) -> Byte Packing1/10
  Header/2(second) -> Byte Packing1/2
  Header/15(reserved) -> Byte Packing1/15
  Clock/1 -> Header/3(time)
  Header/14(recstatus) -> Byte Packing1/14
  Header/6(type) -> Byte Packing1/6
  Header/5(id) -> Byte Packing1/5
  Header/3(third) -> Byte Packing1/3
  Header/16(version) -> Byte Packing1/16
  Header/13(ms) -> Byte Packing1/13
  Header/11(timestatus) -> Byte Packing1/11
  Vector Concatenate1/1 -> Vector Concatenate/1, CRC32/1(data)
  Byte Packing/1 -> Vector Concatenate1/2, Width2/1
  Width5/1 -> UDP Send1/2, UDP Send5/2
  Clock1/1 -> Byte Packing/2
  GNSS Week/1 -> Byte Packing/1
  GPS Origin in llh/1 -> tcs2llhT/4(origin)
  tcs2llhT/3(hgt) -> Byte Packing/5
  Bus Selector/1 -> tcs2llhT/1(x)  "<x_Loc1_m>"
  Bus Selector/2 -> tcs2llhT/2(y)  "<y_Loc1_m>"
  Bus Selector/3 -> tcs2llhT/3(z)  "<z_Loc1_m>"
  Bus Selector/4 -> Byte Packing/6  "<vx_CoGVel1_mps>"
  Bus Selector/5 -> Byte Packing/7  "<vy_CoGVel1_mps>"
  Bus Selector/6 -> Byte Packing/9  "<dPhi_RollRateIMU1_radps>"
  Bus Selector/7 -> Byte Packing/10  "<dTheta_PitchRateIMU1_radps>"
  Constant/1 -> Byte Packing/12
  Constant1/1 -> Byte Packing/8
  grid conv angle/1(gamma) -> Plus/1
  Gain/1 -> Plus/2
  tcs2llhT/2(lon) -> grid conv angle/2(lon), Byte Packing/4
  normalizeAngle360/1(y) -> Byte Packing/11
  Plus/1 -> normalizeAngle360/1(u)
  Angle Conversion2/1 -> Gain/1
  tcs2llhT/1(lat) -> grid conv angle/1(lat), Byte Packing/3
  SimRealState/1 -> Bus Selector1/1
  Bus Selector1/1 -> Angle Conversion2/1  "<psi_rad>"
  Vector Concatenate/1 -> UDP Send1/1, UDP Send5/1, Width5/1

== system controller_dev_sg_HIL_noTP/UDP to Sensors (GNSS, IMU)7/PSRDOP2 ==
  Enable : EnablePort
  Byte Packing : xpcutilitieslib/Byte Packing   MaskPackedDataType=uint8  MaskUnpackedDataTypes={ 'single', 'single', 'single', 'single', 'uint32', 'uint32', 'single', 'uint32', 'single'}  MaskAlignment=1
  Byte Packing1 : xpcutilitieslib/Byte Packing   MaskPackedDataType=uint8  MaskUnpackedDataTypes={'uint8', 'uint8', 'uint8', 'uint8', 'uint16', 'uint8', 'uint8', 'uint16', 'uint16', 'uint8', 'uint8', 'uint16', 'uint32', 'uint32', 'uint16', 'uint16'}  MaskAlignment=1
  CRC32 : MATLAB Function  TreatAsAtomicUnit=on
  Clock : Clock
  GALILEO : Constant  Value=2  OutDataTypeStr=uint32
  GALILEO TDOP : Constant  Value=1.0  OutDataTypeStr=single
  GDOP : Constant  Value=1.0  OutDataTypeStr=single
  GPS : Constant  Value=0  OutDataTypeStr=uint32
  GPS TDOP : Constant  Value=1.0  OutDataTypeStr=single
  HDOP : Constant  Value=1.0  OutDataTypeStr=single
  Header : MATLAB Function  TreatAsAtomicUnit=on
  Message ID : Constant  Value=1163  OutDataTypeStr=uint16
  PDOP : Constant  Value=1.0  OutDataTypeStr=single
  Systems : Constant  Value=2  OutDataTypeStr=uint32
  UDP Send1 : xpcrtudplib/UDP Send  ipAddressVal=10.0.0.20  localPort=40784  toAddress=10.0.0.18  toPort=ModSens_GpsSenDat_SendPort + 1  sampleTime=-1
      settings: SourceProductName=Simulink Real-Time  SourceProductBaseCode=XP
  UDP Send4 : xpcrtudplib/UDP Send  ipAddressVal=10.0.0.20  localPort=40684  toAddress=10.0.0.18  toPort=ModSens_GpsSenDat_SendPort  sampleTime=-1
      settings: SourceProductName=Simulink Real-Time  SourceProductBaseCode=XP
  VDOP : Constant  Value=1.0  OutDataTypeStr=single
  Vector Concatenate : Concatenate
  Vector Concatenate1 : Concatenate
  Width2 : Width
  Width4 : Width
  leap seconds : Constant  Value=19  OutDataTypeStr=single
  uint32touint8 : xpcutilitieslib/Byte Packing   MaskPackedDataType=uint8  MaskUnpackedDataTypes={'uint32'}  MaskAlignment=1
  wires:
  CRC32/1(crc) -> uint32touint8/1
  uint32touint8/1 -> Vector Concatenate/2
  Message ID/1 -> Header/1("id ")
  Header/16(version) -> Byte Packing1/16
  Header/3(third) -> Byte Packing1/3
  Header/14(recstatus) -> Byte Packing1/14
  Clock/1 -> Header/3(time)
  Header/15(reserved) -> Byte Packing1/15
  Header/10(idletime) -> Byte Packing1/10
  Header/13(ms) -> Byte Packing1/13
  Header/2(second) -> Byte Packing1/2
  Header/8(mlength) -> Byte Packing1/8
  Header/11(timestatus) -> Byte Packing1/11
  Header/4(hlength) -> Byte Packing1/4
  Header/1(first) -> Byte Packing1/1
  Header/12(week) -> Byte Packing1/12
  Header/6(type) -> Byte Packing1/6
  leap seconds/1 -> Header/4(leapseconds)
  Header/9(seq) -> Byte Packing1/9
  Header/7(port) -> Byte Packing1/7
  Width2/1 -> Header/2(length)
  Byte Packing1/1 -> Vector Concatenate1/1
  Header/5(id) -> Byte Packing1/5
  GDOP/1 -> Byte Packing/1
  PDOP/1 -> Byte Packing/2
  HDOP/1 -> Byte Packing/3
  VDOP/1 -> Byte Packing/4
  Systems/1 -> Byte Packing/5
  GPS/1 -> Byte Packing/6
  GPS TDOP/1 -> Byte Packing/7
  GALILEO/1 -> Byte Packing/8
  GALILEO TDOP/1 -> Byte Packing/9
  Vector Concatenate1/1 -> Vector Concatenate/1, CRC32/1(data)
  Byte Packing/1 -> Width2/1, Vector Concatenate1/2
  Vector Concatenate/1 -> UDP Send1/1, UDP Send4/1, Width4/1
  Width4/1 -> UDP Send1/2, UDP Send4/2

== system controller_dev_sg_HIL_noTP/UDP to Sensors (GNSS, IMU)7/RAWIMU ==
  VehicleSensorData : Inport
  Enable : EnablePort
  Bus Selector : BusSelector  OutputSignals=az_CoGIMU1_mps2,ay_CoGIMU1_mps2,ax_CoGIMU1_mps2,dPsi_YawRateIMU1_radps,dTheta_PitchRateIMU1_radps,dPhi_RollRateIMU1_radps
  Byte Packing : xpcutilitieslib/Byte Packing   MaskPackedDataType=uint8  MaskUnpackedDataTypes={'uint32', 'double', 'uint32', 'int32', 'int32', 'int32', 'int32', 'int32', 'int32'}  MaskAlignment=1
  Byte Packing1 : xpcutilitieslib/Byte Packing   MaskPackedDataType=uint8  MaskUnpackedDataTypes={'uint8', 'uint8', 'uint8', 'uint8', 'uint16', 'uint16', 'uint32'}  MaskAlignment=1
  CRC32 : MATLAB Function  TreatAsAtomicUnit=on
  Clock : Clock
  Clock1 : Clock
  Constant : Constant  Value=0.200  OutDataTypeStr=double
  Constant1 : Constant  Value=65536  OutDataTypeStr=double
  Constant2 : Constant  Value=0.008  OutDataTypeStr=double
  Constant3 : Constant  Value=1000  OutDataTypeStr=double
  Constant4 : Constant  Value=65536  OutDataTypeStr=double
  Constant6 : Constant  Value=180  OutDataTypeStr=double
  Data Type Conversion{1..6} (6 alike) : DataTypeConversion  OutDataTypeStr=int32
  Data Type Conversion7 : DataTypeConversion  OutDataTypeStr=double
  Data Type Conversion8 : DataTypeConversion  OutDataTypeStr=uint32
  Data Type Conversion9 : DataTypeConversion  OutDataTypeStr=uint32
  DataRate : Constant  Value=125  OutDataTypeStr=double
  DataRate1 : Constant  Value=125  OutDataTypeStr=double
  Divide{,1..20} (21 alike) : Product  Inputs=*/
  GNSS Week : Constant  Value=1900  OutDataTypeStr=uint32
  GNSS Week1 : Constant  Value=1900  OutDataTypeStr=uint16
  Gain1 : Gain  Gain=-1
  Gain2 : Gain  Gain=-1
  IMU Status : Constant  Value=0  OutDataTypeStr=uint32
  Message ID : Constant  Value=325  OutDataTypeStr=uint16
  Message ID1 : Constant  Value=19  OutDataTypeStr=uint8
  Message ID3 : Constant  Value=68  OutDataTypeStr=uint8
  Message ID4 : Constant  Value=170  OutDataTypeStr=uint8
  Message Length : Constant  Value=40  OutDataTypeStr=uint8
  Multiply : Product
  ONE_G : Constant  Value=9.80665  OutDataTypeStr=double
  Pi : Constant  Value=3.14159265358979323846  OutDataTypeStr=double
  UDP Send1 : xpcrtudplib/UDP Send  ipAddressVal=10.0.0.20  localPort=40787  toAddress=10.0.0.18  toPort=ModSens_GpsSenDat_SendPort + 1  sampleTime=-1
      settings: SourceProductName=Simulink Real-Time  SourceProductBaseCode=XP
  UDP Send3 : xpcrtudplib/UDP Send  ipAddressVal=10.0.0.20  localPort=40687  toAddress=10.0.0.18  toPort=ModSens_GpsSenDat_SendPort  sampleTime=-1
      settings: SourceProductName=Simulink Real-Time  SourceProductBaseCode=XP
  Vector Concatenate : Concatenate
  Vector Concatenate1 : Concatenate
  Width3 : Width
  uint32touint8 : xpcutilitieslib/Byte Packing   MaskPackedDataType=uint8  MaskUnpackedDataTypes={'uint32'}  MaskAlignment=1
  wires:
  VehicleSensorData/1 -> Bus Selector/1
  CRC32/1(crc) -> uint32touint8/1
  uint32touint8/1 -> Vector Concatenate/2
  Vector Concatenate1/1 -> Vector Concatenate/1, CRC32/1(data)
  Width3/1 -> UDP Send1/2, UDP Send3/2
  Vector Concatenate/1 -> UDP Send1/1, UDP Send3/1, Width3/1
  Data Type Conversion9/1 -> Byte Packing1/7
  Clock/1 -> Data Type Conversion8/1
  Constant6/1 -> Divide17/2
  Data Type Conversion7/1 -> Byte Packing/2
  Clock1/1 -> Data Type Conversion9/1
  Data Type Conversion6/1 -> Byte Packing/9
  Divide16/1 -> Divide20/1
  GNSS Week/1 -> Byte Packing/1
  Data Type Conversion5/1 -> Byte Packing/8
  Message ID4/1 -> Byte Packing1/1
  Divide17/1 -> Divide20/2, Divide19/2, Divide18/2
  GNSS Week1/1 -> Byte Packing1/6
  Divide1/1 -> Divide6/1
  Divide19/1 -> Data Type Conversion6/1
  Data Type Conversion8/1 -> Data Type Conversion7/1
  Constant3/1 -> Divide4/2
  Message ID/1 -> Byte Packing1/5
  Data Type Conversion2/1 -> Byte Packing/5
  Constant4/1 -> Divide9/2
  Message Length/1 -> Byte Packing1/4
  Divide14/1 -> Divide18/1
  Data Type Conversion1/1 -> Byte Packing/4
  Divide12/1 -> Divide15/1
  Message ID3/1 -> Byte Packing1/2
  DataRate1/1 -> Divide14/2, Divide15/2, Divide16/2, Divide10/2
  Divide5/1 -> Divide3/2, Divide2/2, Divide1/2
  Data Type Conversion3/1 -> Byte Packing/6
  Divide6/1 -> Data Type Conversion1/1
  Multiply/1 -> Divide5/1
  Divide9/1 -> Divide10/1
  Divide11/1 -> Divide14/1
  Divide10/1 -> Divide11/2, Divide12/2, Divide13/2
  Message ID1/1 -> Byte Packing1/3
  Pi/1 -> Divide17/1
  Constant1/1 -> Divide/2
  Constant/1 -> Divide/1
  DataRate/1 -> Divide8/2, Divide7/2, Divide6/2, Divide5/2
  Constant2/1 -> Divide9/1
  Divide18/1 -> Data Type Conversion4/1
  Divide3/1 -> Divide8/1
  Divide/1 -> Multiply/2
  Data Type Conversion4/1 -> Byte Packing/7
  Divide15/1 -> Divide19/1
  Divide2/1 -> Divide7/1
  ONE_G/1 -> Divide4/1
  IMU Status/1 -> Byte Packing/3
  Divide4/1 -> Multiply/1
  Divide13/1 -> Divide16/1
  Byte Packing1/1 -> Vector Concatenate1/1
  Byte Packing/1 -> Vector Concatenate1/2
  Bus Selector/6 -> Divide13/1  "<dPhi_RollRateIMU1_radps>"
  Bus Selector/5 -> Divide12/1  "<dTheta_PitchRateIMU1_radps>"
  Bus Selector/4 -> Divide11/1  "<dPsi_YawRateIMU1_radps>"
  Bus Selector/3 -> Gain2/1  "<ax_CoGIMU1_mps2>"
  Bus Selector/2 -> Gain1/1  "<ay_CoGIMU1_mps2>"
  Bus Selector/1 -> Divide1/1  "<az_CoGIMU1_mps2>"
  Divide20/1 -> Data Type Conversion5/1
  Divide8/1 -> Data Type Conversion2/1
  Divide7/1 -> Data Type Conversion3/1
  Gain1/1 -> Divide2/1
  Gain2/1 -> Divide3/1

== system controller_dev_sg_HIL_noTP/UDP to Sensors (GNSS, IMU)7/Subsystem ==
  Compare To Constant : simulink/Logic and Bit Operations/Compare To Constant  relop=>=  const=1/sensors_freq_gps  OutDataTypeStr=boolean
  Constant6 : Constant  Value=tSPhysics
  Sum : Sum  Inputs=|++
  Switch : Switch  Criteria=u2 > Threshold
  Unit Delay : UnitDelay  SampleTime=-1
  send_gps : Outport
  wires:
  Switch/1 -> Unit Delay/1
  Constant6/1 -> Switch/1, Sum/1
  Compare To Constant/1 -> send_gps/1, Switch/2
  Unit Delay/1 -> Sum/2, Compare To Constant/1
  Sum/1 -> Switch/3

== system controller_dev_sg_HIL_noTP/UDP to Sensors (GNSS, IMU)7/Subsystem1 ==
  Compare To Constant : simulink/Logic and Bit Operations/Compare To Constant  relop=>=  const=1/sensors_freq_imu  OutDataTypeStr=boolean
  Constant6 : Constant  Value=tSPhysics
  Sum : Sum  Inputs=|++
  Switch : Switch  Criteria=u2 > Threshold
  Unit Delay : UnitDelay  SampleTime=-1
  send_imu : Outport
  wires:
  Switch/1 -> Unit Delay/1
  Constant6/1 -> Switch/1, Sum/1
  Compare To Constant/1 -> send_imu/1, Switch/2
  Unit Delay/1 -> Sum/2, Compare To Constant/1
  Sum/1 -> Switch/3

== matlab function controller_dev_sg_HIL_noTP/EnvironmentSim_Communication/prepare data for sending1/normalieAngle1 ==
  data: u input; y output
function y = fcn(u)

y = normalizeAngle(u);

== matlab function controller_dev_sg_HIL_noTP/EnvironmentSim_Communication/prepare data for sending1/normalieAngle2 ==
  data: u input; y output
function y = fcn(u)

y = normalizeAngle(u);

== matlab function controller_dev_sg_HIL_noTP/EnvironmentSim_Communication/prepare data for sending/normalieAngle1 ==
  data: u input; y output
function y = fcn(u)

y = normalizeAngle(u);

== matlab function controller_dev_sg_HIL_noTP/EnvironmentSim_Communication/prepare data for sending/normalieAngle2 ==
  data: u input; y output
function y = fcn(u)

y = normalizeAngle(u);

== matlab function controller_dev_sg_HIL_noTP/EnvironmentSim_Communication/prepare data for sending2/normalieAngle1 ==
  data: u input; y output
function y = fcn(u)

y = normalizeAngle(u);

== matlab function controller_dev_sg_HIL_noTP/EnvironmentSim_Communication/prepare data for sending2/normalieAngle2 ==
  data: u input; y output
function y = fcn(u)

y = normalizeAngle(u);

== matlab function controller_dev_sg_HIL_noTP/EnvironmentSim_Communication/prepare data for sending3/normalieAngle1 ==
  data: u input; y output
function y = fcn(u)

y = normalizeAngle(u);

== matlab function controller_dev_sg_HIL_noTP/EnvironmentSim_Communication/prepare data for sending3/normalieAngle2 ==
  data: u input; y output
function y = fcn(u)

y = normalizeAngle(u);

== matlab function controller_dev_sg_HIL_noTP/EnvironmentSim_Communication/prepare data for sending4/normalieAngle1 ==
  data: u input; y output
function y = fcn(u)

y = normalizeAngle(u);

== matlab function controller_dev_sg_HIL_noTP/EnvironmentSim_Communication/prepare data for sending4/normalieAngle2 ==
  data: u input; y output
function y = fcn(u)

y = normalizeAngle(u);

== matlab function controller_dev_sg_HIL_noTP/EnvironmentSim_Communication/prepare data for sending5/normalieAngle1 ==
  data: u input; y output
function y = fcn(u)

y = normalizeAngle(u);

== matlab function controller_dev_sg_HIL_noTP/EnvironmentSim_Communication/prepare data for sending5/normalieAngle2 ==
  data: u input; y output
function y = fcn(u)

y = normalizeAngle(u);

== matlab function controller_dev_sg_HIL_noTP/EnvironmentSim_Communication/prepare data for sending6/normalieAngle1 ==
  data: u input; y output
function y = fcn(u)

y = normalizeAngle(u);

== matlab function controller_dev_sg_HIL_noTP/EnvironmentSim_Communication/prepare data for sending6/normalieAngle2 ==
  data: u input; y output
function y = fcn(u)

y = normalizeAngle(u);

== matlab function controller_dev_sg_HIL_noTP/EnvironmentSim_Communication/prepare data for sending7/normalieAngle1 ==
  data: u input; y output
function y = fcn(u)

y = normalizeAngle(u);

== matlab function controller_dev_sg_HIL_noTP/EnvironmentSim_Communication/prepare data for sending7/normalieAngle2 ==
  data: u input; y output
function y = fcn(u)

y = normalizeAngle(u);

== matlab function controller_dev_sg_HIL_noTP/EnvironmentSim_Communication/prepare data for sending8/normalieAngle1 ==
  data: u input; y output
function y = fcn(u)

y = normalizeAngle(u);

== matlab function controller_dev_sg_HIL_noTP/EnvironmentSim_Communication/prepare data for sending8/normalieAngle2 ==
  data: u input; y output
function y = fcn(u)

y = normalizeAngle(u);

== matlab function controller_dev_sg_HIL_noTP/EnvironmentSim_Communication/prepare data for sending9/normalieAngle1 ==
  data: u input; y output
function y = fcn(u)

y = normalizeAngle(u);

== matlab function controller_dev_sg_HIL_noTP/EnvironmentSim_Communication/prepare data for sending9/normalieAngle2 ==
  data: u input; y output
function y = fcn(u)

y = normalizeAngle(u);

== matlab function controller_dev_sg_HIL_noTP/UDP to Sensors (GNSS, IMU)/BESTPOS/CRC32 ==
  data: data input; crc output
function crc = fcn(data)

crc = crc32(data);

== matlab function controller_dev_sg_HIL_noTP/UDP to Sensors (GNSS, IMU)/BESTPOS/Header ==
  data: id input; first output; length input; time input; leapseconds input; second output; third output; hlength output; id output; type output; port output; mlength output; seq output; idletime output; timestatus output; week output; ms output; recstatus output; reserved output; version output
function [first, second, third, hlength, id, type, port, mlength, seq, idletime, timestatus, week, ms, recstatus, reserved, version] = fcn(id, length, time, leapseconds)

[first, second, third, hlength, id, type, port, mlength, seq, idletime, timestatus, week, ms, recstatus, reserved, version] = novatel_header(id, length, time, leapseconds);

== matlab function controller_dev_sg_HIL_noTP/UDP to Sensors (GNSS, IMU)/BESTPOS/tcs2llhT ==
  data: x input; lat output; y input; z input; origin input; lon output; hgt output
function [lat, lon, hgt]= fcn(x, y, z, origin)

llh =tcs2llhT([x; y; z], origin);
lat = llh(1,:);
lon = llh(2,:);
hgt = llh(3,:);
end

== matlab function controller_dev_sg_HIL_noTP/UDP to Sensors (GNSS, IMU)/BESTUTM/CRC32 ==
  data: data input; crc output
function crc = fcn(data)

crc = crc32(data);

== matlab function controller_dev_sg_HIL_noTP/UDP to Sensors (GNSS, IMU)/BESTUTM/Header ==
  data: id input; first output; length input; time input; leapseconds input; second output; third output; hlength output; id output; type output; port output; mlength output; seq output; idletime output; timestatus output; week output; ms output; recstatus output; reserved output; version output
function [first, second, third, hlength, id, type, port, mlength, seq, idletime, timestatus, week, ms, recstatus, reserved, version] = fcn(id, length, time, leapseconds)

[first, second, third, hlength, id, type, port, mlength, seq, idletime, timestatus, week, ms, recstatus, reserved, version] = novatel_header(id, length, time, leapseconds);
